simulink model "task19_8"  (R2021a)
settings: Solver=VariableStepAuto  StartTime=0.0  StopTime=10.0  RelTol=1e-3
libraries: simulink x1
settings Model: Creator=reemb  LastModifiedBy=reemb

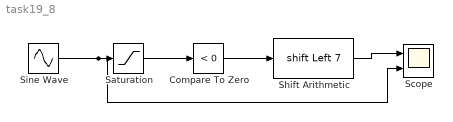
== system task19_8 ==
  Compare To Zero : simulink/Logic and Bit Operations/Compare To Zero  relop=<  OutDataTypeStr=uint8
  Saturation : Saturate  UpperLimit=5  LowerLimit=-5
  Scope : Scope  NumInputPorts=2
  Shift Arithmetic : ArithShift  BitShiftNumber=7  BitShiftDirection=Left
  Sine Wave : Sin  SampleTime=0
  wires:
  Sine Wave/1 -> Scope/2, Saturation/1
  Compare To Zero/1 -> Shift Arithmetic/1
  Saturation/1 -> Compare To Zero/1
  Shift Arithmetic/1 -> Scope/1
